simulink model "EEL_5661_F21_Bicycle_OL_ver3_algebraic_092021"  (R2019a)
settings: Solver=VariableStepAuto  StartTime=0.0  StopTime=6  RelTol=1e-3
libraries: simulink x1
settings Model: Creator=rothz  LastModifiedBy=rothz

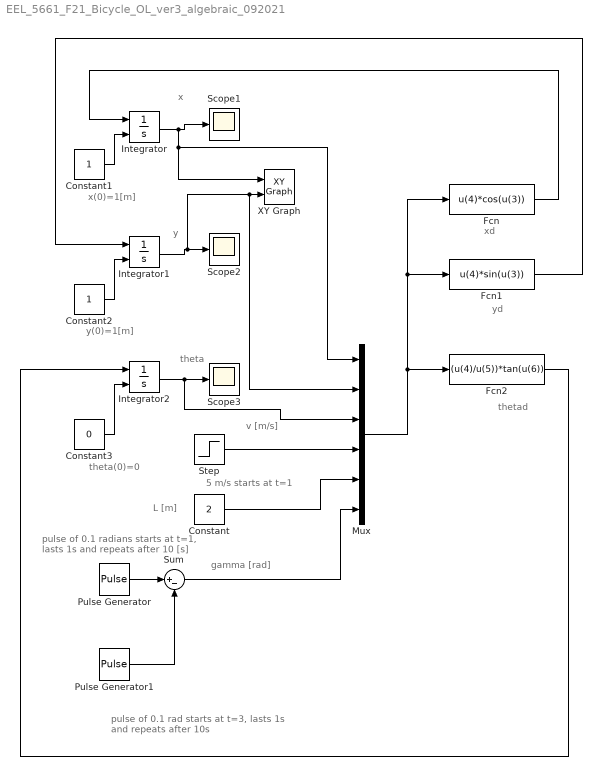
== system EEL_5661_F21_Bicycle_OL_ver3_algebraic_092021 ==
  note: thetad
  note: yd
  note: xd
  note: 5 m/s starts at t=1
  note: v [m/s]
  note: gamma [rad]
  note: pulse of 0.1 rad starts
      | at t=3, lasts 1s and repeats after 10s
  note: pulse of 0.1 radians starts
      | at t=1, lasts 1s and repeats after
      | 10 [s]
  note: theta(0)=0
  note: y(0)=1[m]
  note: x(0)=1[m]
  note: L [m]
  note: theta
  note: y
  note: x
  Constant : Constant  Value=2
  Constant1 : Constant
  Constant2 : Constant
  Constant3 : Constant  Value=0
  Fcn : Fcn  Expr=u(4)*cos(u(3))
  Fcn1 : Fcn  Expr=u(4)*sin(u(3))
  Fcn2 : Fcn  Expr=(u(4)/u(5))*tan(u(6))
  Integrator : Integrator  InitialConditionSource=external
  Integrator1 : Integrator  InitialConditionSource=external
  Integrator2 : Integrator  InitialConditionSource=external
  Mux : Mux  Inputs=6
  Pulse Generator : DiscretePulseGenerator  PulseType=Time based  Amplitude=0.2  Period=10  PulseWidth=10  PhaseDelay=1
  Pulse Generator1 : DiscretePulseGenerator  PulseType=Time based  Amplitude=0.2  Period=10  PulseWidth=10  PhaseDelay=3
  Scope1 : Scope
  Scope2 : Scope
  Scope3 : Scope
  Step : Step  After=5  SampleTime=0
  Sum : Sum  Inputs=|+-
  XY Graph : simulink/Sinks/XY Graph  xmin=-1  xmax=20  ymin=-1  ymax=20  st=-1
  wires:
  Integrator2/1 -> Mux/3, Scope3/1
  Constant3/1 -> Integrator2/2
  Constant2/1 -> Integrator1/2
  Constant1/1 -> Integrator/2
  Integrator/1 -> Mux/1, XY Graph/1, Scope1/1
  Integrator1/1 -> Mux/2, XY Graph/2, Scope2/1
  Pulse Generator1/1 -> Sum/2
  Pulse Generator/1 -> Sum/1
  Step/1 -> Mux/4
  Constant/1 -> Mux/5
  Sum/1 -> Mux/6
  Mux/1 -> Fcn/1, Fcn1/1, Fcn2/1
  Fcn/1 -> Integrator/1
  Fcn1/1 -> Integrator1/1
  Fcn2/1 -> Integrator2/1
